simulink model "gm_uz_pmsm_model_9ph_vnl"  (R2021a)
settings: Solver=FixedStepAuto  StartTime=0.0  StopTime=.5  RelTol=1e-3
PreLoadFcn:
  | uz_pmsm_model_init_parameter
undefined symbols (not defined in the file or in its folder): c, friction_coefficient, inertia, k_i_d, k_p_d, k_p_q, L_d, L_o1, L_o2, L_q, L_x1, L_x2, L_y1, L_y2, L_zero, polepair, psi_pm, R_1, static_friction_torque, ts
libraries: hdlmdlgenlib x220, hdlsllib x18, simulink x11, pid_lib x2
(part 3 of 4)

== system gm_uz_pmsm_model_9ph_vnl/uz_pmsm_model_9ph/Data Type Conversion12 ==
  In1 : Inport
  Data Type Conversion12 : DataTypeConversion  OutDataTypeStr=double  RndMeth=Nearest  SampleTime=1e-08
  Out1 : Outport
  wires:
  Data Type Conversion12/1 -> Out1/1
  In1/1 -> Data Type Conversion12/1

== system gm_uz_pmsm_model_9ph_vnl/uz_pmsm_model_9ph/Data Type Conversion13 ==
  In1 : Inport
  Data Type Conversion13 : DataTypeConversion  OutDataTypeStr=double  RndMeth=Nearest  SampleTime=1e-08
  Out1 : Outport
  wires:
  Data Type Conversion13/1 -> Out1/1
  In1/1 -> Data Type Conversion13/1

== system gm_uz_pmsm_model_9ph_vnl/uz_pmsm_model_9ph/Data Type Conversion15 ==
  In1 : Inport
  Data Type Conversion15 : DataTypeConversion  OutDataTypeStr=single  RndMeth=Nearest  SampleTime=1e-08
  Out1 : Outport
  wires:
  Data Type Conversion15/1 -> Out1/1
  In1/1 -> Data Type Conversion15/1

== system gm_uz_pmsm_model_9ph_vnl/uz_pmsm_model_9ph/Data Type Conversion16 ==
  In1 : Inport
  Data Type Conversion16 : DataTypeConversion  OutDataTypeStr=single  RndMeth=Nearest  SampleTime=1e-08
  Out1 : Outport
  wires:
  Data Type Conversion16/1 -> Out1/1
  In1/1 -> Data Type Conversion16/1

== system gm_uz_pmsm_model_9ph_vnl/uz_pmsm_model_9ph/Data Type Conversion17 ==
  In1 : Inport
  Data Type Conversion17 : DataTypeConversion  OutDataTypeStr=single  RndMeth=Nearest  SampleTime=1e-08
  Out1 : Outport
  wires:
  Data Type Conversion17/1 -> Out1/1
  In1/1 -> Data Type Conversion17/1

== system gm_uz_pmsm_model_9ph_vnl/uz_pmsm_model_9ph/Data Type Conversion18 ==
  In1 : Inport
  Data Type Conversion18 : DataTypeConversion  OutDataTypeStr=single  RndMeth=Nearest  SampleTime=1e-08
  Out1 : Outport
  wires:
  Data Type Conversion18/1 -> Out1/1
  In1/1 -> Data Type Conversion18/1

== system gm_uz_pmsm_model_9ph_vnl/uz_pmsm_model_9ph/Data Type Conversion19 ==
  In1 : Inport
  Data Type Conversion19 : DataTypeConversion  OutDataTypeStr=double  RndMeth=Nearest  SampleTime=1e-08
  Out1 : Outport
  wires:
  Data Type Conversion19/1 -> Out1/1
  In1/1 -> Data Type Conversion19/1

== system gm_uz_pmsm_model_9ph_vnl/uz_pmsm_model_9ph/Data Type Conversion2 ==
  In1 : Inport
  Data Type Conversion2 : DataTypeConversion  OutDataTypeStr=double  RndMeth=Nearest  SampleTime=1e-08
  Out1 : Outport
  wires:
  Data Type Conversion2/1 -> Out1/1
  In1/1 -> Data Type Conversion2/1

== system gm_uz_pmsm_model_9ph_vnl/uz_pmsm_model_9ph/Data Type Conversion21 ==
  In1 : Inport
  Data Type Conversion21 : DataTypeConversion  OutDataTypeStr=double  RndMeth=Nearest  SampleTime=1e-08
  Out1 : Outport
  wires:
  Data Type Conversion21/1 -> Out1/1
  In1/1 -> Data Type Conversion21/1

== system gm_uz_pmsm_model_9ph_vnl/uz_pmsm_model_9ph/Data Type Conversion26 ==
  In1 : Inport
  Data Type Conversion26 : DataTypeConversion  OutDataTypeStr=single  RndMeth=Nearest  SampleTime=1e-08
  Out1 : Outport
  wires:
  Data Type Conversion26/1 -> Out1/1
  In1/1 -> Data Type Conversion26/1

== system gm_uz_pmsm_model_9ph_vnl/uz_pmsm_model_9ph/Data Type Conversion3 ==
  In1 : Inport
  Data Type Conversion3 : DataTypeConversion  OutDataTypeStr=double  RndMeth=Nearest  SampleTime=1e-08
  Out1 : Outport
  wires:
  Data Type Conversion3/1 -> Out1/1
  In1/1 -> Data Type Conversion3/1

== system gm_uz_pmsm_model_9ph_vnl/uz_pmsm_model_9ph/Data Type Conversion30 ==
  In1 : Inport
  Data Type Conversion30 : DataTypeConversion  OutDataTypeStr=single  RndMeth=Nearest  SampleTime=1e-08
  Out1 : Outport
  wires:
  Data Type Conversion30/1 -> Out1/1
  In1/1 -> Data Type Conversion30/1

== system gm_uz_pmsm_model_9ph_vnl/uz_pmsm_model_9ph/Data Type Conversion31 ==
  In1 : Inport
  Data Type Conversion31 : DataTypeConversion  OutDataTypeStr=fixdt(1, 25, 12)  RndMeth=Nearest  SampleTime=1e-08
  Out1 : Outport
  wires:
  Data Type Conversion31/1 -> Out1/1
  In1/1 -> Data Type Conversion31/1

== system gm_uz_pmsm_model_9ph_vnl/uz_pmsm_model_9ph/Data Type Conversion32 ==
  In1 : Inport
  Data Type Conversion32 : DataTypeConversion  OutDataTypeStr=double  RndMeth=Nearest  SampleTime=1e-08
  Out1 : Outport
  wires:
  Data Type Conversion32/1 -> Out1/1
  In1/1 -> Data Type Conversion32/1

== system gm_uz_pmsm_model_9ph_vnl/uz_pmsm_model_9ph/Data Type Conversion4 ==
  In1 : Inport
  Data Type Conversion4 : DataTypeConversion  OutDataTypeStr=double  RndMeth=Nearest  SampleTime=1e-08
  Out1 : Outport
  wires:
  Data Type Conversion4/1 -> Out1/1
  In1/1 -> Data Type Conversion4/1

== system gm_uz_pmsm_model_9ph_vnl/uz_pmsm_model_9ph/Data Type Conversion41 ==
  In1 : Inport
  Data Type Conversion41 : DataTypeConversion  OutDataTypeStr=double  RndMeth=Nearest  SampleTime=1e-08
  Out1 : Outport
  wires:
  Data Type Conversion41/1 -> Out1/1
  In1/1 -> Data Type Conversion41/1

== system gm_uz_pmsm_model_9ph_vnl/uz_pmsm_model_9ph/Data Type Conversion5 ==
  In1 : Inport
  Data Type Conversion5 : DataTypeConversion  OutDataTypeStr=double  RndMeth=Nearest  SampleTime=1e-08
  Out1 : Outport
  wires:
  Data Type Conversion5/1 -> Out1/1
  In1/1 -> Data Type Conversion5/1

== system gm_uz_pmsm_model_9ph_vnl/uz_pmsm_model_9ph/Data Type Conversion51 ==
  In1 : Inport
  Data Type Conversion51 : DataTypeConversion  OutDataTypeStr=double  RndMeth=Nearest  SampleTime=1e-08
  Out1 : Outport
  wires:
  Data Type Conversion51/1 -> Out1/1
  In1/1 -> Data Type Conversion51/1

== system gm_uz_pmsm_model_9ph_vnl/uz_pmsm_model_9ph/Data Type Conversion6 ==
  In1 : Inport
  Data Type Conversion6 : DataTypeConversion  OutDataTypeStr=single  RndMeth=Nearest  SampleTime=1e-08
  Out1 : Outport
  wires:
  Data Type Conversion6/1 -> Out1/1
  In1/1 -> Data Type Conversion6/1

== system gm_uz_pmsm_model_9ph_vnl/uz_pmsm_model_9ph/Data Type Conversion61 ==
  In1 : Inport
  Data Type Conversion61 : DataTypeConversion  OutDataTypeStr=double  RndMeth=Nearest  SampleTime=1e-08
  Out1 : Outport
  wires:
  Data Type Conversion61/1 -> Out1/1
  In1/1 -> Data Type Conversion61/1

== system gm_uz_pmsm_model_9ph_vnl/uz_pmsm_model_9ph/Data Type Conversion71 ==
  In1 : Inport
  Data Type Conversion71 : DataTypeConversion  OutDataTypeStr=double  RndMeth=Nearest  SampleTime=1e-08
  Out1 : Outport
  wires:
  Data Type Conversion71/1 -> Out1/1
  In1/1 -> Data Type Conversion71/1

== system gm_uz_pmsm_model_9ph_vnl/uz_pmsm_model_9ph/Data Type Conversion8 ==
  In1 : Inport
  Data Type Conversion8 : DataTypeConversion  OutDataTypeStr=double  RndMeth=Nearest  SampleTime=1e-08
  Out1 : Outport
  wires:
  Data Type Conversion8/1 -> Out1/1
  In1/1 -> Data Type Conversion8/1

== system gm_uz_pmsm_model_9ph_vnl/uz_pmsm_model_9ph/Data Type Conversion9 ==
  In1 : Inport
  Data Type Conversion9 : DataTypeConversion  OutDataTypeStr=double  RndMeth=Nearest  SampleTime=1e-08
  Out1 : Outport
  wires:
  Data Type Conversion9/1 -> Out1/1
  In1/1 -> Data Type Conversion9/1

== system gm_uz_pmsm_model_9ph_vnl/uz_pmsm_model_9ph/Data Type Conversion91 ==
  In1 : Inport
  Data Type Conversion91 : DataTypeConversion  OutDataTypeStr=double  RndMeth=Nearest  SampleTime=1e-08
  Out1 : Outport
  wires:
  Data Type Conversion91/1 -> Out1/1
  In1/1 -> Data Type Conversion91/1

== system gm_uz_pmsm_model_9ph_vnl/uz_pmsm_model_9ph/Divide ==
  In1 : Inport
  In2 : Inport  Port=2
  Divide : Product  Inputs=**  OutDataTypeStr=double  SampleTime=1e-08
  Out1 : Outport
  wires:
  Divide/1 -> Out1/1
  In2/1 -> Divide/2
  In1/1 -> Divide/1

== system gm_uz_pmsm_model_9ph_vnl/uz_pmsm_model_9ph/Divide1 ==
  In1 : Inport
  In2 : Inport  Port=2
  Divide1 : Product  Inputs=*/  OutDataTypeStr=double  SampleTime=1e-08
  Out1 : Outport
  wires:
  Divide1/1 -> Out1/1
  In2/1 -> Divide1/2
  In1/1 -> Divide1/1

== system gm_uz_pmsm_model_9ph_vnl/uz_pmsm_model_9ph/Divide10 ==
  In1 : Inport
  In2 : Inport  Port=2
  Divide10 : Product  Inputs=**  OutDataTypeStr=double  SampleTime=1e-08
  Out1 : Outport
  wires:
  Divide10/1 -> Out1/1
  In2/1 -> Divide10/2
  In1/1 -> Divide10/1

== system gm_uz_pmsm_model_9ph_vnl/uz_pmsm_model_9ph/Divide11 ==
  In1 : Inport
  In2 : Inport  Port=2
  Divide11 : Product  Inputs=*/  OutDataTypeStr=double  SampleTime=1e-08
  Out1 : Outport
  wires:
  Divide11/1 -> Out1/1
  In2/1 -> Divide11/2
  In1/1 -> Divide11/1

== system gm_uz_pmsm_model_9ph_vnl/uz_pmsm_model_9ph/Divide12 ==
  In1 : Inport
  In2 : Inport  Port=2
  Divide12 : Product  Inputs=**  OutDataTypeStr=double  SampleTime=1e-08
  Out1 : Outport
  wires:
  Divide12/1 -> Out1/1
  In2/1 -> Divide12/2
  In1/1 -> Divide12/1

== system gm_uz_pmsm_model_9ph_vnl/uz_pmsm_model_9ph/Divide13 ==
  In1 : Inport
  In2 : Inport  Port=2
  Divide13 : Product  Inputs=*/  OutDataTypeStr=double  SampleTime=1e-08
  Out1 : Outport
  wires:
  Divide13/1 -> Out1/1
  In2/1 -> Divide13/2
  In1/1 -> Divide13/1

== system gm_uz_pmsm_model_9ph_vnl/uz_pmsm_model_9ph/Divide14 ==
  In1 : Inport
  In2 : Inport  Port=2
  Divide14 : Product  Inputs=**  OutDataTypeStr=double  SampleTime=1e-08
  Out1 : Outport
  wires:
  Divide14/1 -> Out1/1
  In2/1 -> Divide14/2
  In1/1 -> Divide14/1

== system gm_uz_pmsm_model_9ph_vnl/uz_pmsm_model_9ph/Divide2 ==
  In1 : Inport
  In2 : Inport  Port=2
  Divide2 : Product  Inputs=**  OutDataTypeStr=double  SampleTime=1e-08
  Out1 : Outport
  wires:
  Divide2/1 -> Out1/1
  In2/1 -> Divide2/2
  In1/1 -> Divide2/1

== system gm_uz_pmsm_model_9ph_vnl/uz_pmsm_model_9ph/Divide3 ==
  In1 : Inport
  In2 : Inport  Port=2
  Divide3 : Product  Inputs=*/  OutDataTypeStr=double  SampleTime=1e-08
  Out1 : Outport
  wires:
  Divide3/1 -> Out1/1
  In2/1 -> Divide3/2
  In1/1 -> Divide3/1

== system gm_uz_pmsm_model_9ph_vnl/uz_pmsm_model_9ph/Divide4 ==
  In1 : Inport
  In2 : Inport  Port=2
  Divide4 : Product  Inputs=**  OutDataTypeStr=double  SampleTime=1e-08
  Out1 : Outport
  wires:
  Divide4/1 -> Out1/1
  In2/1 -> Divide4/2
  In1/1 -> Divide4/1

== system gm_uz_pmsm_model_9ph_vnl/uz_pmsm_model_9ph/Divide5 ==
  In1 : Inport
  In2 : Inport  Port=2
  Divide5 : Product  Inputs=*/  OutDataTypeStr=double  SampleTime=1e-08
  Out1 : Outport
  wires:
  Divide5/1 -> Out1/1
  In2/1 -> Divide5/2
  In1/1 -> Divide5/1

== system gm_uz_pmsm_model_9ph_vnl/uz_pmsm_model_9ph/Divide6 ==
  In1 : Inport
  In2 : Inport  Port=2
  Divide6 : Product  Inputs=**  OutDataTypeStr=double  SampleTime=1e-08
  Out1 : Outport
  wires:
  Divide6/1 -> Out1/1
  In2/1 -> Divide6/2
  In1/1 -> Divide6/1

== system gm_uz_pmsm_model_9ph_vnl/uz_pmsm_model_9ph/Divide7 ==
  In1 : Inport
  In2 : Inport  Port=2
  Divide7 : Product  Inputs=*/  OutDataTypeStr=double  SampleTime=1e-08
  Out1 : Outport
  wires:
  Divide7/1 -> Out1/1
  In2/1 -> Divide7/2
  In1/1 -> Divide7/1

== system gm_uz_pmsm_model_9ph_vnl/uz_pmsm_model_9ph/Divide8 ==
  In1 : Inport
  In2 : Inport  Port=2
  Divide8 : Product  Inputs=**  OutDataTypeStr=double  SampleTime=1e-08
  Out1 : Outport
  wires:
  Divide8/1 -> Out1/1
  In2/1 -> Divide8/2
  In1/1 -> Divide8/1

== system gm_uz_pmsm_model_9ph_vnl/uz_pmsm_model_9ph/Divide9 ==
  In1 : Inport
  In2 : Inport  Port=2
  Divide9 : Product  Inputs=*/  OutDataTypeStr=double  SampleTime=1e-08
  Out1 : Outport
  wires:
  Divide9/1 -> Out1/1
  In2/1 -> Divide9/2
  In1/1 -> Divide9/1

== system gm_uz_pmsm_model_9ph_vnl/uz_pmsm_model_9ph/Factor ==
  In1 : Inport
  In2 : Inport  Port=2
  Factor : Product  Inputs=**  OutDataTypeStr=double  SampleTime=1e-08
  Out1 : Outport
  wires:
  Factor/1 -> Out1/1
  In2/1 -> Factor/2
  In1/1 -> Factor/1

== system gm_uz_pmsm_model_9ph_vnl/uz_pmsm_model_9ph/Gain ==
  In1 : Inport
  In2 : Inport  Port=2
  Gain : Product  Inputs=**  OutDataTypeStr=double  SampleTime=1e-08
  Out1 : Outport
  wires:
  Gain/1 -> Out1/1
  In2/1 -> Gain/2
  In1/1 -> Gain/1

== system gm_uz_pmsm_model_9ph_vnl/uz_pmsm_model_9ph/Gain1 ==
  In1 : Inport
  In2 : Inport  Port=2
  Gain1 : Product  Inputs=**  OutDataTypeStr=double  SampleTime=1e-08
  Out1 : Outport
  wires:
  Gain1/1 -> Out1/1
  In2/1 -> Gain1/2
  In1/1 -> Gain1/1

== system gm_uz_pmsm_model_9ph_vnl/uz_pmsm_model_9ph/Gain10 ==
  In1 : Inport
  In2 : Inport  Port=2
  Gain10 : Product  Inputs=**  OutDataTypeStr=double  SampleTime=1e-08
  Out1 : Outport
  wires:
  Gain10/1 -> Out1/1
  In2/1 -> Gain10/2
  In1/1 -> Gain10/1

== system gm_uz_pmsm_model_9ph_vnl/uz_pmsm_model_9ph/Gain2 ==
  In1 : Inport
  In2 : Inport  Port=2
  Gain2 : Product  Inputs=**  OutDataTypeStr=double  SampleTime=1e-08
  Out1 : Outport
  wires:
  Gain2/1 -> Out1/1
  In2/1 -> Gain2/2
  In1/1 -> Gain2/1

== system gm_uz_pmsm_model_9ph_vnl/uz_pmsm_model_9ph/Gain3 ==
  In1 : Inport
  In2 : Inport  Port=2
  Gain3 : Product  Inputs=**  OutDataTypeStr=double  SampleTime=1e-08
  Out1 : Outport
  wires:
  Gain3/1 -> Out1/1
  In2/1 -> Gain3/2
  In1/1 -> Gain3/1

== system gm_uz_pmsm_model_9ph_vnl/uz_pmsm_model_9ph/Gain4 ==
  In1 : Inport
  In2 : Inport  Port=2
  Gain4 : Product  Inputs=**  OutDataTypeStr=double  SampleTime=1e-08
  Out1 : Outport
  wires:
  Gain4/1 -> Out1/1
  In2/1 -> Gain4/2
  In1/1 -> Gain4/1

== system gm_uz_pmsm_model_9ph_vnl/uz_pmsm_model_9ph/Gain5 ==
  In1 : Inport
  In2 : Inport  Port=2
  Gain5 : Product  Inputs=**  OutDataTypeStr=double  SampleTime=1e-08
  Out1 : Outport
  wires:
  Gain5/1 -> Out1/1
  In2/1 -> Gain5/2
  In1/1 -> Gain5/1

== system gm_uz_pmsm_model_9ph_vnl/uz_pmsm_model_9ph/Gain6 ==
  In1 : Inport
  In2 : Inport  Port=2
  Gain6 : Product  Inputs=**  OutDataTypeStr=double  SampleTime=1e-08
  Out1 : Outport
  wires:
  Gain6/1 -> Out1/1
  In2/1 -> Gain6/2
  In1/1 -> Gain6/1

== system gm_uz_pmsm_model_9ph_vnl/uz_pmsm_model_9ph/Gain7 ==
  In1 : Inport
  In2 : Inport  Port=2
  Gain7 : Product  Inputs=**  OutDataTypeStr=double  SampleTime=1e-08
  Out1 : Outport
  wires:
  Gain7/1 -> Out1/1
  In2/1 -> Gain7/2
  In1/1 -> Gain7/1

== system gm_uz_pmsm_model_9ph_vnl/uz_pmsm_model_9ph/Gain8 ==
  In1 : Inport
  In2 : Inport  Port=2
  Gain8 : Product  Inputs=**  OutDataTypeStr=double  SampleTime=1e-08
  Out1 : Outport
  wires:
  Gain8/1 -> Out1/1
  In2/1 -> Gain8/2
  In1/1 -> Gain8/1

== system gm_uz_pmsm_model_9ph_vnl/uz_pmsm_model_9ph/Gain9 ==
  In1 : Inport
  In2 : Inport  Port=2
  Gain9 : Product  Inputs=**  OutDataTypeStr=double  SampleTime=1e-08
  Out1 : Outport
  wires:
  Gain9/1 -> Out1/1
  In2/1 -> Gain9/2
  In1/1 -> Gain9/1

== system gm_uz_pmsm_model_9ph_vnl/uz_pmsm_model_9ph/Product ==
  In1 : Inport
  In2 : Inport  Port=2
  Product : Product  Inputs=**  OutDataTypeStr=double  SampleTime=1e-08
  Out1 : Outport
  wires:
  Product/1 -> Out1/1
  In2/1 -> Product/2
  In1/1 -> Product/1

== system gm_uz_pmsm_model_9ph_vnl/uz_pmsm_model_9ph/Product1 ==
  In1 : Inport
  In2 : Inport  Port=2
  Product1 : Product  Inputs=**  OutDataTypeStr=double  SampleTime=1e-08
  Out1 : Outport
  wires:
  Product1/1 -> Out1/1
  In2/1 -> Product1/2
  In1/1 -> Product1/1

== system gm_uz_pmsm_model_9ph_vnl/uz_pmsm_model_9ph/Product10 ==
  In1 : Inport
  In2 : Inport  Port=2
  Product10 : Product  Inputs=**  OutDataTypeStr=double  SampleTime=1e-08
  Out1 : Outport
  wires:
  Product10/1 -> Out1/1
  In2/1 -> Product10/2
  In1/1 -> Product10/1

== system gm_uz_pmsm_model_9ph_vnl/uz_pmsm_model_9ph/Product11 ==
  In1 : Inport
  In2 : Inport  Port=2
  Product11 : Product  Inputs=**  OutDataTypeStr=double  SampleTime=1e-08
  Out1 : Outport
  wires:
  Product11/1 -> Out1/1
  In2/1 -> Product11/2
  In1/1 -> Product11/1

== system gm_uz_pmsm_model_9ph_vnl/uz_pmsm_model_9ph/Product12 ==
  In1 : Inport
  In2 : Inport  Port=2
  Product12 : Product  Inputs=**  OutDataTypeStr=double  SampleTime=1e-08
  Out1 : Outport
  wires:
  Product12/1 -> Out1/1
  In2/1 -> Product12/2
  In1/1 -> Product12/1

== system gm_uz_pmsm_model_9ph_vnl/uz_pmsm_model_9ph/Product2 ==
  In1 : Inport
  In2 : Inport  Port=2
  Product2 : Product  Inputs=**  OutDataTypeStr=double  SampleTime=1e-08
  Out1 : Outport
  wires:
  Product2/1 -> Out1/1
  In2/1 -> Product2/2
  In1/1 -> Product2/1

== system gm_uz_pmsm_model_9ph_vnl/uz_pmsm_model_9ph/Product3 ==
  In1 : Inport
  In2 : Inport  Port=2
  Product3 : Product  Inputs=**  OutDataTypeStr=double  SampleTime=1e-08
  Out1 : Outport
  wires:
  Product3/1 -> Out1/1
  In2/1 -> Product3/2
  In1/1 -> Product3/1

== system gm_uz_pmsm_model_9ph_vnl/uz_pmsm_model_9ph/Product4 ==
  In1 : Inport
  In2 : Inport  Port=2
  Product4 : Product  Inputs=**  OutDataTypeStr=double  SampleTime=1e-08
  Out1 : Outport
  wires:
  Product4/1 -> Out1/1
  In2/1 -> Product4/2
  In1/1 -> Product4/1

== system gm_uz_pmsm_model_9ph_vnl/uz_pmsm_model_9ph/Product5 ==
  In1 : Inport
  In2 : Inport  Port=2
  Product5 : Product  Inputs=**  OutDataTypeStr=double  SampleTime=1e-08
  Out1 : Outport
  wires:
  Product5/1 -> Out1/1
  In2/1 -> Product5/2
  In1/1 -> Product5/1

== system gm_uz_pmsm_model_9ph_vnl/uz_pmsm_model_9ph/Product6 ==
  In1 : Inport
  In2 : Inport  Port=2
  Product6 : Product  Inputs=**  OutDataTypeStr=double  SampleTime=1e-08
  Out1 : Outport
  wires:
  Product6/1 -> Out1/1
  In2/1 -> Product6/2
  In1/1 -> Product6/1

== system gm_uz_pmsm_model_9ph_vnl/uz_pmsm_model_9ph/Product7 ==
  In1 : Inport
  In2 : Inport  Port=2
  Product7 : Product  Inputs=**  OutDataTypeStr=double  SampleTime=1e-08
  Out1 : Outport
  wires:
  Product7/1 -> Out1/1
  In2/1 -> Product7/2
  In1/1 -> Product7/1

== system gm_uz_pmsm_model_9ph_vnl/uz_pmsm_model_9ph/Product8 ==
  In1 : Inport
  In2 : Inport  Port=2
  Product8 : Product  Inputs=**  OutDataTypeStr=double  SampleTime=1e-08
  Out1 : Outport
  wires:
  Product8/1 -> Out1/1
  In2/1 -> Product8/2
  In1/1 -> Product8/1

== system gm_uz_pmsm_model_9ph_vnl/uz_pmsm_model_9ph/Product9 ==
  In1 : Inport
  In2 : Inport  Port=2
  Product9 : Product  Inputs=**  OutDataTypeStr=double  SampleTime=1e-08
  Out1 : Outport
  wires:
  Product9/1 -> Out1/1
  In2/1 -> Product9/2
  In1/1 -> Product9/1

== system gm_uz_pmsm_model_9ph_vnl/uz_pmsm_model_9ph/Sign1 ==
  In1 : Inport
  Sign1 : Signum  SampleTime=1e-08
  Out1 : Outport
  wires:
  Sign1/1 -> Out1/1
  In1/1 -> Sign1/1

== system gm_uz_pmsm_model_9ph_vnl/uz_pmsm_model_9ph/Sum ==
  In1 : Inport
  In2 : Inport  Port=2
  Sum : Sum  Inputs=+-  OutDataTypeStr=double  SampleTime=1e-08
  Out1 : Outport
  wires:
  Sum/1 -> Out1/1
  In2/1 -> Sum/2
  In1/1 -> Sum/1

== system gm_uz_pmsm_model_9ph_vnl/uz_pmsm_model_9ph/Sum1 ==
  In1 : Inport
  In2 : Inport  Port=2
  Sum1 : Sum  Inputs=+-  OutDataTypeStr=double  SampleTime=1e-08
  Out1 : Outport
  wires:
  Sum1/1 -> Out1/1
  In2/1 -> Sum1/2
  In1/1 -> Sum1/1

== system gm_uz_pmsm_model_9ph_vnl/uz_pmsm_model_9ph/Sum1_stage2 ==
  In1 : Inport
  In2 : Inport  Port=2
  Sum1_stage2 : Sum  Inputs=+-  OutDataTypeStr=double  SampleTime=1e-08
  Out1 : Outport
  wires:
  Sum1_stage2/1 -> Out1/1
  In2/1 -> Sum1_stage2/2
  In1/1 -> Sum1_stage2/1

== system gm_uz_pmsm_model_9ph_vnl/uz_pmsm_model_9ph/Sum1_stage3 ==
  In1 : Inport
  In2 : Inport  Port=2
  Sum1_stage3 : Sum  Inputs=+-  OutDataTypeStr=double  SampleTime=1e-08
  Out1 : Outport
  wires:
  Sum1_stage3/1 -> Out1/1
  In2/1 -> Sum1_stage3/2
  In1/1 -> Sum1_stage3/1

== system gm_uz_pmsm_model_9ph_vnl/uz_pmsm_model_9ph/Sum2 ==
  In1 : Inport
  In2 : Inport  Port=2
  Sum2 : Sum  Inputs=+-  OutDataTypeStr=double  SampleTime=1e-08
  Out1 : Outport
  wires:
  Sum2/1 -> Out1/1
  In2/1 -> Sum2/2
  In1/1 -> Sum2/1

== system gm_uz_pmsm_model_9ph_vnl/uz_pmsm_model_9ph/Sum3 ==
  In1 : Inport
  In2 : Inport  Port=2
  Sum3 : Sum  OutDataTypeStr=double  SampleTime=1e-08
  Out1 : Outport
  wires:
  Sum3/1 -> Out1/1
  In2/1 -> Sum3/2
  In1/1 -> Sum3/1

== system gm_uz_pmsm_model_9ph_vnl/uz_pmsm_model_9ph/Sum31 ==
  In1 : Inport
  In2 : Inport  Port=2
  Sum31 : Sum  OutDataTypeStr=double  SampleTime=1e-08
  Out1 : Outport
  wires:
  Sum31/1 -> Out1/1
  In2/1 -> Sum31/2
  In1/1 -> Sum31/1

== system gm_uz_pmsm_model_9ph_vnl/uz_pmsm_model_9ph/Sum310 ==
  In1 : Inport
  In2 : Inport  Port=2
  Sum310 : Sum  Inputs=+-  OutDataTypeStr=double  SampleTime=1e-08
  Out1 : Outport
  wires:
  Sum310/1 -> Out1/1
  In2/1 -> Sum310/2
  In1/1 -> Sum310/1

== system gm_uz_pmsm_model_9ph_vnl/uz_pmsm_model_9ph/Sum311 ==
  In1 : Inport
  In2 : Inport  Port=2
  Sum311 : Sum  OutDataTypeStr=double  SampleTime=1e-08
  Out1 : Outport
  wires:
  Sum311/1 -> Out1/1
  In2/1 -> Sum311/2
  In1/1 -> Sum311/1

== system gm_uz_pmsm_model_9ph_vnl/uz_pmsm_model_9ph/Sum32 ==
  In1 : Inport
  In2 : Inport  Port=2
  Sum32 : Sum  OutDataTypeStr=double  SampleTime=1e-08
  Out1 : Outport
  wires:
  Sum32/1 -> Out1/1
  In2/1 -> Sum32/2
  In1/1 -> Sum32/1

== system gm_uz_pmsm_model_9ph_vnl/uz_pmsm_model_9ph/Sum33 ==
  In1 : Inport
  In2 : Inport  Port=2
  Sum33 : Sum  OutDataTypeStr=double  SampleTime=1e-08
  Out1 : Outport
  wires:
  Sum33/1 -> Out1/1
  In2/1 -> Sum33/2
  In1/1 -> Sum33/1

== system gm_uz_pmsm_model_9ph_vnl/uz_pmsm_model_9ph/Sum34 ==
  In1 : Inport
  In2 : Inport  Port=2
  Sum34 : Sum  OutDataTypeStr=double  SampleTime=1e-08
  Out1 : Outport
  wires:
  Sum34/1 -> Out1/1
  In2/1 -> Sum34/2
  In1/1 -> Sum34/1

== system gm_uz_pmsm_model_9ph_vnl/uz_pmsm_model_9ph/Sum35 ==
  In1 : Inport
  In2 : Inport  Port=2
  Sum35 : Sum  OutDataTypeStr=double  SampleTime=1e-08
  Out1 : Outport
  wires:
  Sum35/1 -> Out1/1
  In2/1 -> Sum35/2
  In1/1 -> Sum35/1

== system gm_uz_pmsm_model_9ph_vnl/uz_pmsm_model_9ph/Sum36 ==
  In1 : Inport
  In2 : Inport  Port=2
  Sum36 : Sum  OutDataTypeStr=double  SampleTime=1e-08
  Out1 : Outport
  wires:
  Sum36/1 -> Out1/1
  In2/1 -> Sum36/2
  In1/1 -> Sum36/1

== system gm_uz_pmsm_model_9ph_vnl/uz_pmsm_model_9ph/Sum37 ==
  In1 : Inport
  In2 : Inport  Port=2
  Sum37 : Sum  OutDataTypeStr=double  SampleTime=1e-08
  Out1 : Outport
  wires:
  Sum37/1 -> Out1/1
  In2/1 -> Sum37/2
  In1/1 -> Sum37/1

== system gm_uz_pmsm_model_9ph_vnl/uz_pmsm_model_9ph/Sum38 ==
  In1 : Inport
  In2 : Inport  Port=2
  Sum38 : Sum  OutDataTypeStr=double  SampleTime=1e-08
  Out1 : Outport
  wires:
  Sum38/1 -> Out1/1
  In2/1 -> Sum38/2
  In1/1 -> Sum38/1

== system gm_uz_pmsm_model_9ph_vnl/uz_pmsm_model_9ph/Sum39 ==
  In1 : Inport
  In2 : Inport  Port=2
  Sum39 : Sum  OutDataTypeStr=double  SampleTime=1e-08
  Out1 : Outport
  wires:
  Sum39/1 -> Out1/1
  In2/1 -> Sum39/2
  In1/1 -> Sum39/1

== system gm_uz_pmsm_model_9ph_vnl/uz_pmsm_model_9ph/Sum5 ==
  In1 : Inport
  In2 : Inport  Port=2
  Sum5 : Sum  OutDataTypeStr=double  SampleTime=1e-08
  Out1 : Outport
  wires:
  Sum5/1 -> Out1/1
  In2/1 -> Sum5/2
  In1/1 -> Sum5/1

== system gm_uz_pmsm_model_9ph_vnl/uz_pmsm_model_9ph/Sum_stage2 ==
  In1 : Inport
  In2 : Inport  Port=2
  Sum_stage2 : Sum  Inputs=+-  OutDataTypeStr=double  SampleTime=1e-08
  Out1 : Outport
  wires:
  Sum_stage2/1 -> Out1/1
  In2/1 -> Sum_stage2/2
  In1/1 -> Sum_stage2/1

== system gm_uz_pmsm_model_9ph_vnl/uz_pmsm_model_9ph/Sum_stage3 ==
  In1 : Inport
  In2 : Inport  Port=2
  Sum_stage3 : Sum  OutDataTypeStr=double  SampleTime=1e-08
  Out1 : Outport
  wires:
  Sum_stage3/1 -> Out1/1
  In2/1 -> Sum_stage3/2
  In1/1 -> Sum_stage3/1

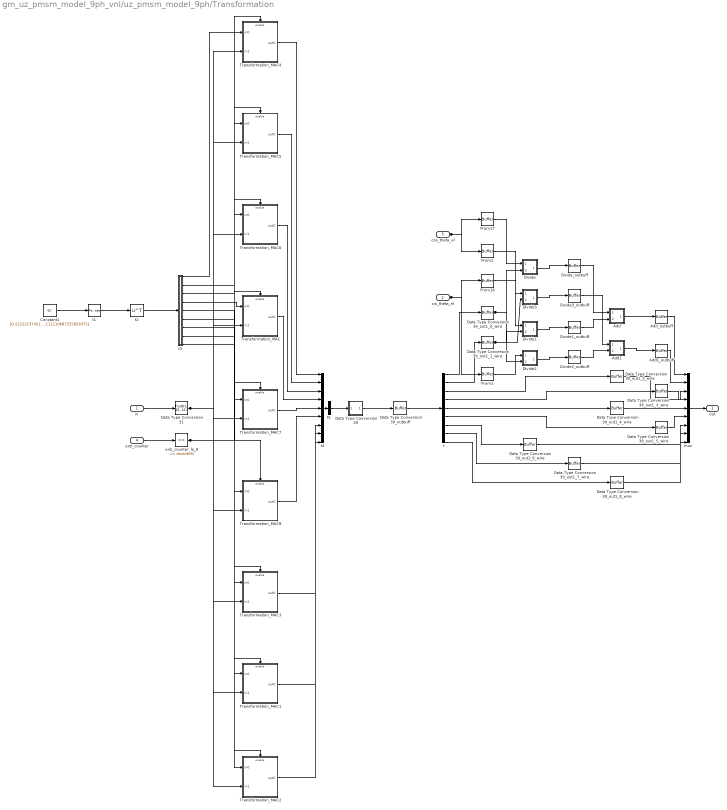
== system gm_uz_pmsm_model_9ph_vnl/uz_pmsm_model_9ph/Transformation ==
  in : Inport  OutDataTypeStr=fixdt(1, 25, 12)  PortDimensions=[9]  SampleTime=1e-08
  sin_theta_el : Inport  Port=2  OutDataTypeStr=single  SampleTime=1e-08
  cos_theta_el : Inport  Port=3  OutDataTypeStr=single  SampleTime=1e-08
  enb_counter : Inport  Port=4  OutDataTypeStr=uint8  SampleTime=1e-08
  Add : Subsystem
      mask Display: disp('NFP\nadd');
  Add1 : Subsystem
      mask Display: disp('NFP\nadd');
  Add1_outbuff : hdlmdlgenlib/Buffer
      settings: SourceProductBaseCode=SL
  Add_outbuff : hdlmdlgenlib/Buffer
      settings: SourceProductBaseCode=SL
  Constant1 : Constant  Value=[0.22222137451171875;0;0.22222137451171875;0;0.22222137451171875;0;0.22222137451171875;0;0.111110687255859375;-0.111110687255859375;0.1924495697021484375;0.22222137451171875;0;-0.111110687255859375;-0.1924495697021484375;-0.111110687255859375;0.1924495697021484375;0.111110687255859375;-0.111110687255859375;-0.1924495697021484375;0.22222137451171875;0;-0.111110687255859375;0.1924495697021484375;-0.111110687255859375;-0.1924495697021484375;0.111110687255859375;0.208820343017578125;0.0760040283203125;0.111110687255859375;0.1924495697021484375;-0.0385875701904296875;0.218845367431640625;-0.1702327728271484375;0.142841339111328125;-0.111110687255859375;-0.1702327728271484375;0.142841339111328125;0.111110687255859375;0.1924495697021484375;0.208820343017578125;-0.0760040283203125;-0.0385875701904296875;-0.218845367431640625;-0.111110687255859375;-0.0385875701904296875;-0.218845367431640625;0.111110687255859375;0.1924495697021484375;-0.1702327728271484375;-0.142841339111328125;0.208820343017578125;0.0760040283203125;-0.111110687255859375;0.1702327728271484375;0.142841339111328125;-0.111110687255859375;0.1924495697021484375;-0.208820343017578125;-0.0760040283203125;0.0385875701904296875;-0.218845367431640625;0.111110687255859375;-0.208820343017578125;0.0760040283203125;-0.111110687255859375;0.1924495697021484375;0.0385875701904296875;0.218845367431640625;0.1702327728271484375;0.142841339111328125;0.111110687255859375;0.0385875701904296875;-0.218845367431640625;-0.111110687255859375;0.1924495697021484375;0.1702327728271484375;-0.142841339111328125;-0.208820343017578125;0.0760040283203125;0.111110687255859375]  OutDataTypeStr=fixdt(1, 18, 19)  SampleTime=1e-08
  Data Type Conversion31 : DataTypeConversion  OutDataTypeStr=fixdt(1, 25, 12)  RndMeth=Nearest  SampleTime=1e-08
  Data Type Conversion39 : Subsystem
      mask Display: disp('NFP\nconv');
  Data Type Conversion39_out1_0_wire : hdlmdlgenlib/Buffer
      settings: SourceProductBaseCode=SL
  Data Type Conversion39_out1_1_wire : hdlmdlgenlib/Buffer
      settings: SourceProductBaseCode=SL
  Data Type Conversion39_out1_2_wire : hdlmdlgenlib/Buffer
      settings: SourceProductBaseCode=SL
  Data Type Conversion39_out1_3_wire : hdlmdlgenlib/Buffer
      settings: SourceProductBaseCode=SL
  Data Type Conversion39_out1_4_wire : hdlmdlgenlib/Buffer
      settings: SourceProductBaseCode=SL
  Data Type Conversion39_out1_5_wire : hdlmdlgenlib/Buffer
      settings: SourceProductBaseCode=SL
  Data Type Conversion39_out1_6_wire : hdlmdlgenlib/Buffer
      settings: SourceProductBaseCode=SL
  Data Type Conversion39_out1_7_wire : hdlmdlgenlib/Buffer
      settings: SourceProductBaseCode=SL
  Data Type Conversion39_out1_8_wire : hdlmdlgenlib/Buffer
      settings: SourceProductBaseCode=SL
  Data Type Conversion39_outbuff : hdlmdlgenlib/Buffer
      settings: SourceProductBaseCode=SL
  Divide : Subsystem
      mask Display: disp('NFP\nmul');
  Divide1 : Subsystem
      mask Display: disp('NFP\nmul');
  Divide1_outbuff : hdlmdlgenlib/Buffer
      settings: SourceProductBaseCode=SL
  Divide2 : Subsystem
      mask Display: disp('NFP\nmul');
  Divide2_outbuff : hdlmdlgenlib/Buffer
      settings: SourceProductBaseCode=SL
  Divide3 : Subsystem
      mask Display: disp('NFP\nmul');
  Divide3_outbuff : hdlmdlgenlib/Buffer
      settings: SourceProductBaseCode=SL
  Divide_outbuff : hdlmdlgenlib/Buffer
      settings: SourceProductBaseCode=SL
  From{1..2,17..18} (4 alike) : hdlmdlgenlib/Buffer
      settings: SourceProductBaseCode=SL
  Transformation_MAC : Subsystem
      settings: MinAlgLoopOccurrences=on
  Transformation_MAC1 : Subsystem
      settings: MinAlgLoopOccurrences=on
  Transformation_MAC2 : Subsystem
      settings: MinAlgLoopOccurrences=on
  Transformation_MAC3 : Subsystem
      settings: MinAlgLoopOccurrences=on
  Transformation_MAC4 : Subsystem
      settings: MinAlgLoopOccurrences=on
  Transformation_MAC5 : Subsystem
      settings: MinAlgLoopOccurrences=on
  Transformation_MAC6 : Subsystem
      settings: MinAlgLoopOccurrences=on
  Transformation_MAC7 : Subsystem
      settings: MinAlgLoopOccurrences=on
  Transformation_MAC8 : Subsystem
      settings: MinAlgLoopOccurrences=on
  enb_counter_le_8 : simulink/Logic and Bit Operations/Compare To Constant  relop=<=  const=double(8)  OutDataTypeStr=boolean
  mux : Mux  Inputs=9
  t : Demux  Outputs=9
  t1 : Reshape  OutputDimensionality=Customize  OutputDimensions=[9,9]
  t2 : Math  Operator=transpose  SaturateOnIntegerOverflow=on
  t3 : Subsystem
  t4 : Mux  Inputs=9
  t5 : Concatenate  NumInputs=1  Mode=Multidimensional array  ConcatenateDimension=2
  out : Outport  SampleTime=1e-08
  wires:
  enb_counter/1 -> enb_counter_le_8/1
  cos_theta_el/1 -> From17/1, From2/1
  sin_theta_el/1 -> From1/1, From18/1
  in/1 -> Data Type Conversion31/1
  enb_counter_le_8/1 -> Transformation_MAC2/Enable, Transformation_MAC1/Enable, Transformation_MAC3/Enable, Transformation_MAC8/Enable, Transformation_MAC7/Enable, Transformation_MAC/Enable, Transformation_MAC6/Enable, Transformation_MAC5/Enable, Transformation_MAC4/Enable
  Divide3/1(Out1) -> Divide3_outbuff/1
  Divide2/1(Out1) -> Divide2_outbuff/1
  Divide1/1(Out1) -> Divide1_outbuff/1
  Divide/1(Out1) -> Divide_outbuff/1
  Data Type Conversion39/1(Out1) -> Data Type Conversion39_outbuff/1
  Add1/1(Out1) -> Add1_outbuff/1
  Add/1(Out1) -> Add_outbuff/1
  From1/1 -> Divide2/1(In1)
  From18/1 -> Divide1/1(In1)
  From2/1 -> Divide3/1(In1)
  From17/1 -> Divide/1(In1)
  t4/1 -> t5/1
  Transformation_MAC2/1(out0) -> t4/9
  Transformation_MAC1/1(out0) -> t4/8
  Transformation_MAC3/1(out0) -> t4/7
  Transformation_MAC8/1(out0) -> t4/6
  Transformation_MAC7/1(out0) -> t4/5
  Transformation_MAC/1(out0) -> t4/4
  Transformation_MAC6/1(out0) -> t4/3
  Transformation_MAC5/1(out0) -> t4/2
  Transformation_MAC4/1(out0) -> t4/1
  t3/9(out8) -> Transformation_MAC2/1(in0)
  t3/8(out7) -> Transformation_MAC1/1(in0)
  t3/7(out6) -> Transformation_MAC3/1(in0)
  t3/6(out5) -> Transformation_MAC8/1(in0)
  t3/5(out4) -> Transformation_MAC7/1(in0)
  t3/4(out3) -> Transformation_MAC/1(in0)
  t3/3(out2) -> Transformation_MAC6/1(in0)
  t3/2(out1) -> Transformation_MAC5/1(in0)
  t3/1(out0) -> Transformation_MAC4/1(in0)
  t2/1 -> t3/1(in0)
  Constant1/1 -> t1/1
  t/9 -> Data Type Conversion39_out1_8_wire/1
  t/8 -> Data Type Conversion39_out1_7_wire/1
  t/7 -> Data Type Conversion39_out1_6_wire/1
  t/6 -> Data Type Conversion39_out1_5_wire/1
  t/5 -> Data Type Conversion39_out1_4_wire/1
  t/4 -> Data Type Conversion39_out1_3_wire/1
  t/3 -> Data Type Conversion39_out1_2_wire/1
  t/2 -> Data Type Conversion39_out1_1_wire/1
  t/1 -> Data Type Conversion39_out1_0_wire/1
  mux/1 -> out/1
  t5/1 -> Data Type Conversion39/1(In1)
  Divide3_outbuff/1 -> Add1/1(In1)
  Divide2_outbuff/1 -> Add1/2(In2)
  Divide1_outbuff/1 -> Add/2(In2)
  Divide_outbuff/1 -> Add/1(In1)
  Data Type Conversion39_out1_8_wire/1 -> mux/9
  Data Type Conversion39_out1_7_wire/1 -> mux/8
  Data Type Conversion39_out1_6_wire/1 -> mux/7
  Data Type Conversion39_out1_5_wire/1 -> mux/6
  Data Type Conversion39_out1_4_wire/1 -> mux/5
  Data Type Conversion39_out1_3_wire/1 -> mux/4
  Data Type Conversion39_out1_2_wire/1 -> mux/3
  Data Type Conversion39_out1_1_wire/1 -> Divide1/2(In2), Divide3/2(In2)
  Data Type Conversion39_out1_0_wire/1 -> Divide/2(In2), Divide2/2(In2)
  Data Type Conversion39_outbuff/1 -> t/1
  Data Type Conversion31/1 -> Transformation_MAC2/2(in1), Transformation_MAC1/2(in1), Transformation_MAC3/2(in1), Transformation_MAC8/2(in1), Transformation_MAC7/2(in1), Transformation_MAC/2(in1), Transformation_MAC6/2(in1), Transformation_MAC5/2(in1), Transformation_MAC4/2(in1)
  t1/1 -> t2/1
  Add1_outbuff/1 -> mux/2
  Add_outbuff/1 -> mux/1

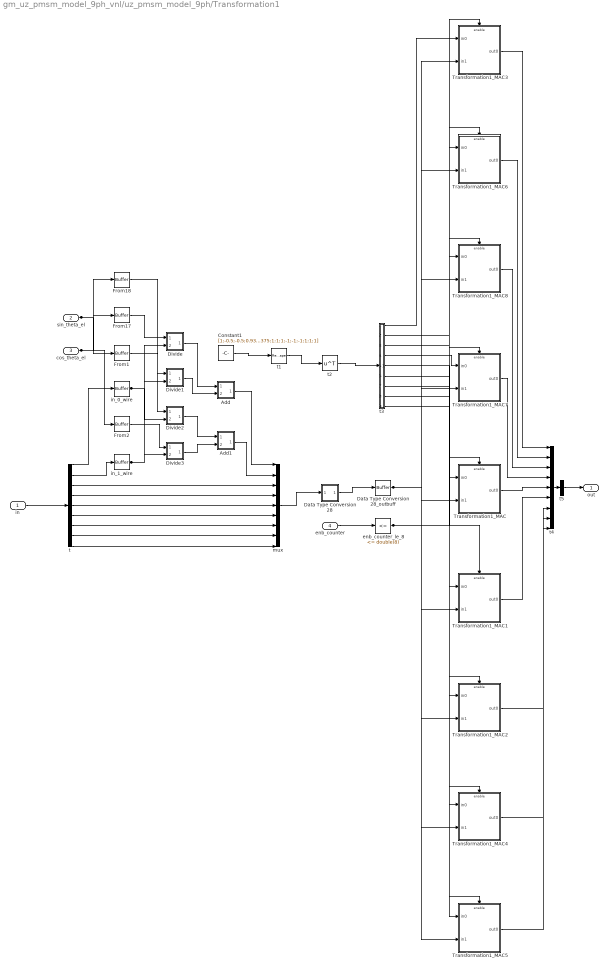
== system gm_uz_pmsm_model_9ph_vnl/uz_pmsm_model_9ph/Transformation1 ==
  in : Inport  OutDataTypeStr=single  PortDimensions=[9]  SampleTime=1e-08
  sin_theta_el : Inport  Port=2  OutDataTypeStr=single  SampleTime=1e-08
  cos_theta_el : Inport  Port=3  OutDataTypeStr=single  SampleTime=1e-08
  enb_counter : Inport  Port=4  OutDataTypeStr=uint8  SampleTime=1e-08
  Add : Subsystem
      mask Display: disp('NFP\nadd');
  Add1 : Subsystem
      mask Display: disp('NFP\nadd');
  Constant1 : Constant  Value=[1;-0.5;-0.5;0.939697265625;-0.7660369873046875;-0.17364501953125;0.7660369873046875;-0.939697265625;0.17364501953125;0;0.86602783203125;-0.86602783203125;0.3420257568359375;0.642791748046875;-0.98480224609375;0.642791748046875;0.3420257568359375;-0.98480224609375;1;1;1;0.5;0.5;0.5;-0.5;-0.5;-0.5;0;0;0;0.86602783203125;0.86602783203125;0.86602783203125;0.86602783203125;0.86602783203125;0.86602783203125;1;-0.5;-0.5;-0.17364501953125;0.939697265625;-0.7660369873046875;-0.939697265625;0.17364501953125;0.7660369873046875;0;-0.86602783203125;0.86602783203125;0.98480224609375;-0.3420257568359375;-0.642791748046875;-0.3420257568359375;0.98480224609375;-0.642791748046875;1;-0.5;-0.5;-0.7660369873046875;-0.17364501953125;0.939697265625;0.17364501953125;0.7660369873046875;-0.939697265625;0;0.86602783203125;-0.86602783203125;0.642791748046875;-0.98480224609375;0.3420257568359375;-0.98480224609375;0.642791748046875;0.3420257568359375;1;1;1;-1;-1;-1;1;1;1]  OutDataTypeStr=fixdt(1, 18, 16)  SampleTime=1e-08
  Data Type Conversion28 : Subsystem
      mask Display: disp('NFP\nconv');
  Data Type Conversion28_outbuff : hdlmdlgenlib/Buffer
      settings: SourceProductBaseCode=SL
  Divide : Subsystem
      mask Display: disp('NFP\nmul');
  Divide1 : Subsystem
      mask Display: disp('NFP\nmul');
  Divide2 : Subsystem
      mask Display: disp('NFP\nmul');
  Divide3 : Subsystem
      mask Display: disp('NFP\nmul');
  From{1..2,17..18} (4 alike) : hdlmdlgenlib/Buffer
      settings: SourceProductBaseCode=SL
  Transformation1_MAC : Subsystem
      settings: MinAlgLoopOccurrences=on
  Transformation1_MAC1 : Subsystem
      settings: MinAlgLoopOccurrences=on
  Transformation1_MAC2 : Subsystem
      settings: MinAlgLoopOccurrences=on
  Transformation1_MAC3 : Subsystem
      settings: MinAlgLoopOccurrences=on
  Transformation1_MAC4 : Subsystem
      settings: MinAlgLoopOccurrences=on
  Transformation1_MAC5 : Subsystem
      settings: MinAlgLoopOccurrences=on
  Transformation1_MAC6 : Subsystem
      settings: MinAlgLoopOccurrences=on
  Transformation1_MAC7 : Subsystem
      settings: MinAlgLoopOccurrences=on
  Transformation1_MAC8 : Subsystem
      settings: MinAlgLoopOccurrences=on
  enb_counter_le_8 : simulink/Logic and Bit Operations/Compare To Constant  relop=<=  const=double(8)  OutDataTypeStr=boolean
  in_0_wire : hdlmdlgenlib/Buffer
      settings: SourceProductBaseCode=SL
  in_1_wire : hdlmdlgenlib/Buffer
      settings: SourceProductBaseCode=SL
  mux : Mux  Inputs=9
  t : Demux  Outputs=9
  t1 : Reshape  OutputDimensionality=Customize  OutputDimensions=[9,9]
  t2 : Math  Operator=transpose  SaturateOnIntegerOverflow=on
  t3 : Subsystem
  t4 : Mux  Inputs=9
  t5 : Concatenate  NumInputs=1  Mode=Multidimensional array  ConcatenateDimension=2
  out : Outport  SampleTime=1e-08
  wires:
  enb_counter/1 -> enb_counter_le_8/1
  cos_theta_el/1 -> From17/1, From2/1
  sin_theta_el/1 -> From1/1, From18/1
  in/1 -> t/1
  enb_counter_le_8/1 -> Transformation1_MAC5/Enable, Transformation1_MAC4/Enable, Transformation1_MAC2/Enable, Transformation1_MAC1/Enable, Transformation1_MAC/Enable, Transformation1_MAC7/Enable, Transformation1_MAC8/Enable, Transformation1_MAC6/Enable, Transformation1_MAC3/Enable
  Divide3/1(Out1) -> Add1/2(In2)
  Divide2/1(Out1) -> Add1/1(In1)
  Divide1/1(Out1) -> Add/2(In2)
  Divide/1(Out1) -> Add/1(In1)
  Data Type Conversion28/1(Out1) -> Data Type Conversion28_outbuff/1
  Add1/1(Out1) -> mux/2
  Add/1(Out1) -> mux/1
  t4/1 -> t5/1
  Transformation1_MAC5/1(out0) -> t4/9
  Transformation1_MAC4/1(out0) -> t4/8
  Transformation1_MAC2/1(out0) -> t4/7
  Transformation1_MAC1/1(out0) -> t4/6
  Transformation1_MAC/1(out0) -> t4/5
  Transformation1_MAC7/1(out0) -> t4/4
  Transformation1_MAC8/1(out0) -> t4/3
  Transformation1_MAC6/1(out0) -> t4/2
  Transformation1_MAC3/1(out0) -> t4/1
  t3/9(out8) -> Transformation1_MAC5/1(in0)
  t3/8(out7) -> Transformation1_MAC4/1(in0)
  t3/7(out6) -> Transformation1_MAC2/1(in0)
  t3/6(out5) -> Transformation1_MAC1/1(in0)
  t3/5(out4) -> Transformation1_MAC/1(in0)
  t3/4(out3) -> Transformation1_MAC7/1(in0)
  t3/3(out2) -> Transformation1_MAC8/1(in0)
  t3/2(out1) -> Transformation1_MAC6/1(in0)
  t3/1(out0) -> Transformation1_MAC3/1(in0)
  t2/1 -> t3/1(in0)
  Constant1/1 -> t1/1
  t/9 -> mux/9
  t/8 -> mux/8
  t/7 -> mux/7
  t/6 -> mux/6
  t/5 -> mux/5
  t/4 -> mux/4
  t/3 -> mux/3
  t/2 -> in_1_wire/1
  t/1 -> in_0_wire/1
  mux/1 -> Data Type Conversion28/1(In1)
  t5/1 -> out/1
  From2/1 -> Divide3/1(In1)
  From18/1 -> Divide1/1(In1)
  From17/1 -> Divide/1(In1)
  From1/1 -> Divide2/1(In1)
  in_1_wire/1 -> Divide1/2(In2), Divide3/2(In2)
  in_0_wire/1 -> Divide/2(In2), Divide2/2(In2)
  Data Type Conversion28_outbuff/1 -> Transformation1_MAC5/2(in1), Transformation1_MAC4/2(in1), Transformation1_MAC2/2(in1), Transformation1_MAC1/2(in1), Transformation1_MAC/2(in1), Transformation1_MAC7/2(in1), Transformation1_MAC8/2(in1), Transformation1_MAC6/2(in1), Transformation1_MAC3/2(in1)
  t1/1 -> t2/1

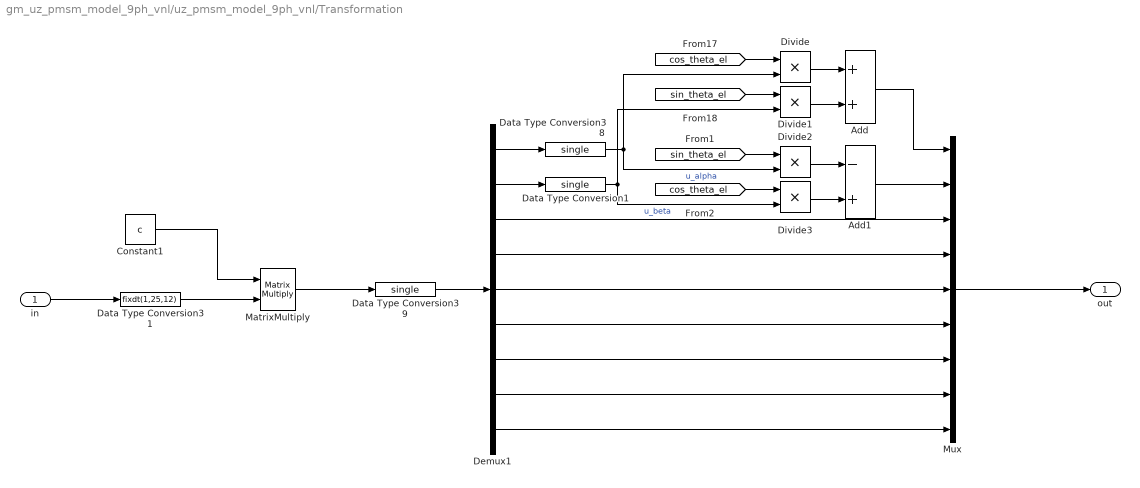
== system gm_uz_pmsm_model_9ph_vnl/uz_pmsm_model_9ph_vnl/Transformation ==
  in : Inport
  Add : Sum
  Add1 : Sum  Inputs=-+
  Constant1 : Constant  Value=c  OutDataTypeStr=fixdt(1,18)  SampleTime=-1
  Data Type Conversion1 : DataTypeConversion  OutDataTypeStr=single  RndMeth=Nearest
  Data Type Conversion31 : DataTypeConversion  OutDataTypeStr=fixdt(1,25,12)  RndMeth=Nearest
  Data Type Conversion38 : DataTypeConversion  OutDataTypeStr=single  RndMeth=Nearest
  Data Type Conversion39 : DataTypeConversion  OutDataTypeStr=single  RndMeth=Nearest
  Demux1 : Demux  Outputs=9
  Divide{,1..3} (4 alike) : Product  Inputs=**
  MatrixMultiply : Product  Multiplication=Matrix(*)
  Mux : Mux  Inputs=9
  out : Outport
  wires:
  Data Type Conversion31/1 -> MatrixMultiply/2
  in/1 -> Data Type Conversion31/1
  Data Type Conversion39/1 -> Demux1/1
  Constant1/1 -> MatrixMultiply/1
  MatrixMultiply/1 -> Data Type Conversion39/1
  Divide2/1 -> Add1/1
  Divide3/1 -> Add1/2
  [cos_theta_el] -> Divide3/1
  [sin_theta_el] -> Divide2/1
  [cos_theta_el] -> Divide/1
  [sin_theta_el] -> Divide1/1
  Divide1/1 -> Add/2
  Divide/1 -> Add/1
  Data Type Conversion1/1 -> Divide3/2, Divide1/2  "u_beta"
  Data Type Conversion38/1 -> Divide2/2, Divide/2  "u_alpha"
  Add/1 -> Mux/1
  Add1/1 -> Mux/2
  Demux1/2 -> Data Type Conversion1/1
  Demux1/1 -> Data Type Conversion38/1
  Mux/1 -> out/1
  Demux1/9 -> Mux/9
  Demux1/8 -> Mux/8
  Demux1/7 -> Mux/7
  Demux1/6 -> Mux/6
  Demux1/5 -> Mux/5
  Demux1/4 -> Mux/4
  Demux1/3 -> Mux/3

== system gm_uz_pmsm_model_9ph_vnl/uz_pmsm_model_9ph_vnl/Transformation1 ==
  in : Inport
  Add : Sum  Inputs=+-
  Add1 : Sum
  Constant1 : Constant  Value=inv(c)  OutDataTypeStr=fixdt(1,18)  SampleTime=-1
  Data Type Conversion28 : DataTypeConversion  OutDataTypeStr=fixdt(1,25,12)  RndMeth=Nearest
  Demux1 : Demux  Outputs=9
  Divide{,1..3} (4 alike) : Product  Inputs=**
  MatrixMultiply : Product  Multiplication=Matrix(*)
  Mux : Mux  Inputs=9
  out : Outport
  wires:
  MatrixMultiply/1 -> out/1
  Constant1/1 -> MatrixMultiply/1
  Data Type Conversion28/1 -> MatrixMultiply/2
  Add1/1 -> Mux/2
  [cos_theta_el] -> Divide3/1
  Divide2/1 -> Add1/1
  [sin_theta_el] -> Divide2/1
  Divide3/1 -> Add1/2
  Demux1/1 -> Divide/2, Divide2/2  "i_d"
  Divide1/1 -> Add/2
  [cos_theta_el] -> Divide/1
  Divide/1 -> Add/1
  Add/1 -> Mux/1
  Demux1/2 -> Divide1/2, Divide3/2  "i_q"
  [sin_theta_el] -> Divide1/1
  Demux1/7 -> Mux/7
  Demux1/9 -> Mux/9
  Demux1/5 -> Mux/5
  Demux1/3 -> Mux/3
  Demux1/4 -> Mux/4
  Demux1/6 -> Mux/6
  Demux1/8 -> Mux/8
  Mux/1 -> Data Type Conversion28/1
  in/1 -> Demux1/1

== system gm_uz_pmsm_model_9ph_vnl/uz_pmsm_model_9ph_vnl/integrator1 ==
  in : Inport
  reset : Inport  Port=2
  Delay1 : Delay  DelayLength=1  ExternalReset=Level
      settings: InputPortMap=u0,r5
  Gain : Gain  Gain=ts  OutDataTypeStr=double
  Sum3 : Sum  Inputs=|++  OutDataTypeStr=double
  outt : Outport
  wires:
  in/1 -> Gain/1
  Gain/1 -> Sum3/1
  reset/1 -> Delay1/2
  Delay1/1 -> Sum3/2, outt/1
  Sum3/1 -> Delay1/1

== system gm_uz_pmsm_model_9ph_vnl/uz_pmsm_model_9ph_vnl/mechanical_system ==
  note: This delay breaks the algebraic loop between mechanical and electrical system.
      | Introduces a delay of 500ns.
  reset : Inport
  M_Mi : Inport  Port=2
  mu : Inport  Port=3
  M_n0 : Inport  Port=4
  reciprocal_J : Inport  Port=5
  load_torque : Inport  Port=6
  Abs : Abs
  Delay : Delay  DelayLength=1
  Product11 : Product
  Product12 : Product
  Product4 : Product
  Sign1 : Signum
  Sum : Sum  Inputs=|+-
  Sum1 : Sum  Inputs=|+-
  Sum5 : Sum  Inputs=|++
  integrator1 : Subsystem
  omega_mech : Outport
  wires:
  Delay/1 -> Sum1/1
  Product4/1 -> Sum/2
  Sum/1 -> Delay/1
  load_torque/1 -> Sum1/2
  Sum1/1 -> Product11/2
  M_Mi/1 -> Sum/1
  reciprocal_J/1 -> Product11/1
  M_n0/1 -> Sum5/2
  mu/1 -> Product12/1
  Product12/1 -> Sum5/1
  reset/1 -> integrator1/1(reset)
  Abs/1 -> Product12/2
  integrator1/1(outt) -> omega_mech/1, Abs/1, Sign1/1
  Sign1/1 -> Product4/2
  Sum5/1 -> Product4/1
  Product11/1 -> integrator1/2(in)

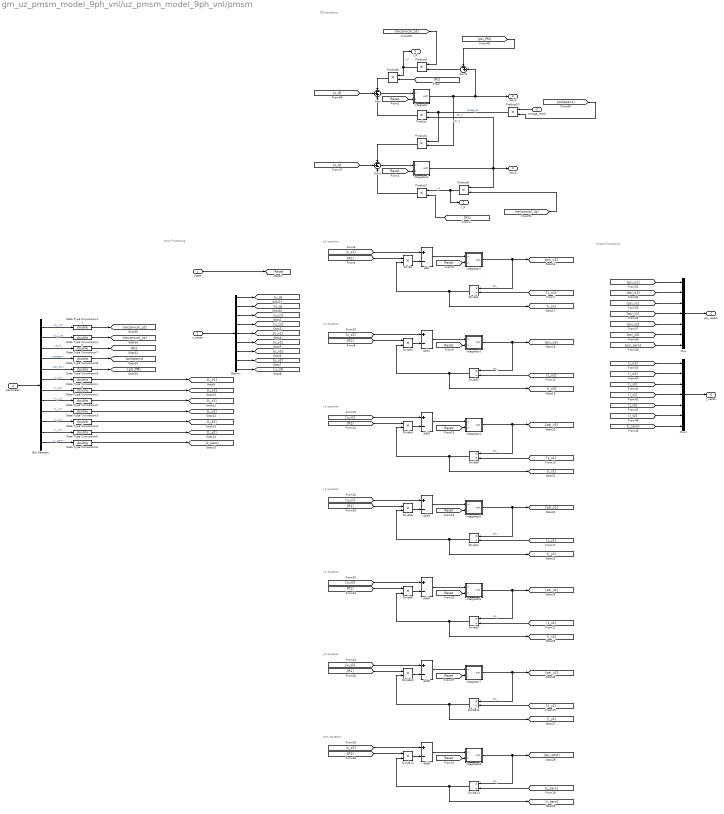
== system gm_uz_pmsm_model_9ph_vnl/uz_pmsm_model_9ph_vnl/pmsm ==
  note: Output Processing
  note: zero equation
  note: y2 equation
  note: x2 equation
  note: y1 equation
  note: x1 equation
  note: o2 equation
  note: DQ equations
  note: o1 equation
  note: Input Processing
  reset : Inport
  u_vector : Inport  Port=2
  omega_mech : Inport  Port=3
  parameter : Inport  Port=4
  Add{,1..6} (7 alike) : Sum  Inputs=+-
  Bus Selector : BusSelector  OutputSignals=1_L_d,1_L_q,R_1,polepair,psi_pm,L_o1,L_o2,L_x1,L_y1,L_x2,L_y2,L_zero
  Data Type Conversion{1..12} (12 alike) : DataTypeConversion  OutDataTypeStr=double  RndMeth=Nearest
  Demux : Demux  Outputs=9
  Divide{,2,4,6,8,10,12} (7 alike) : Product  Inputs=**
  Divide{1,3,5,7,9,11,13} (7 alike) : Product  Inputs=*/
  Mux : Mux  Inputs=7
  Mux1 : Mux  Inputs=7
  Product{,1,5..8,10} (7 alike) : Product
  Sum : Sum  Inputs=-++
  Sum1 : Sum  Inputs=-+-
  Sum2 : Sum  Inputs=-+|
  integrator : Subsystem
  integrator1 : Subsystem
  integrator2 : Subsystem
  integrator3 : Subsystem
  integrator4 : Subsystem
  integrator5 : Subsystem
  integrator6 : Subsystem
  integrator7 : Subsystem
  integrator8 : Subsystem
  I_d : Outport
  I_q : Outport  Port=2
  psi_d : Outport  Port=3
  psi_q : Outport  Port=4
  psi_vector : Outport  Port=5
  I_vector : Outport  Port=6
  tag scope: Reset=global
  wires:
  [R1] -> Divide6/1
  Data Type Conversion11/1 -> [reciprocal_Ld]
  Data Type Conversion12/1 -> [reciprocal_Lq]
  [reciprocal_Lq] -> Product6/2
  Data Type Conversion9/1 -> [psi_PM]
  Data Type Conversion8/1 -> [polepairs]
  Bus Selector/1 -> Data Type Conversion11/1  "<1_L_d>"
  Bus Selector/2 -> Data Type Conversion12/1  "<1_L_q>"
  Bus Selector/5 -> Data Type Conversion9/1  "<psi_pm>"
  Bus Selector/4 -> Data Type Conversion8/1  "<polepair>"
  Data Type Conversion7/1 -> [R1]
  Bus Selector/3 -> Data Type Conversion7/1  "<R_1>"
  Data Type Conversion6/1 -> [L_zero]
  Data Type Conversion5/1 -> [L_y2]
  Data Type Conversion4/1 -> [L_x2]
  Data Type Conversion3/1 -> [L_y1]
  Data Type Conversion2/1 -> [L_x1]
  Data Type Conversion1/1 -> [L_o2]
  Data Type Conversion10/1 -> [L_o1]
  Bus Selector/6 -> Data Type Conversion10/1  "<L_o1>"
  Bus Selector/7 -> Data Type Conversion1/1  "<L_o2>"
  Bus Selector/8 -> Data Type Conversion2/1  "<L_x1>"
  Bus Selector/9 -> Data Type Conversion3/1  "<L_y1>"
  Bus Selector/10 -> Data Type Conversion4/1  "<L_x2>"
  Bus Selector/11 -> Data Type Conversion5/1  "<L_y2>"
  Bus Selector/12 -> Data Type Conversion6/1  "<L_zero>"
  parameter/1 -> Bus Selector/1
  Demux/2 -> [u_q]
  Demux/1 -> [u_d]
  Demux/3 -> [u_z1]
  Demux/4 -> [u_z2]
  Demux/5 -> [u_x1]
  Demux/6 -> [u_y1]
  Demux/7 -> [u_x2]
  Demux/8 -> [u_y2]
  Demux/9 -> [u_z3]
  [i_zero] -> Mux1/7
  [i_y2] -> Mux1/6
  [i_x2] -> Mux1/5
  [i_y1] -> Mux1/4
  [i_x1] -> Mux1/3
  [i_o2] -> Mux1/2
  [psi_zero] -> Mux/7
  [psi_y2] -> Mux/6
  [psi_x2] -> Mux/5
  [psi_y1] -> Mux/4
  [psi_x1] -> Mux/3
  [psi_o2] -> Mux/2
  [i_o1] -> Mux1/1
  [psi_o1] -> Mux/1
  Mux1/1 -> I_vector/1
  Mux/1 -> psi_vector/1
  integrator8/1(outt) -> Divide13/1, [psi_zero]  "psi_"
  [R1] -> Divide12/1
  Add6/1 -> integrator8/1(in)
  Divide12/1 -> Add6/2
  Divide13/1 -> Divide12/2, [i_zero]
  [u_z3] -> Add6/1
  [L_zero] -> Divide13/2
  [Reset] -> integrator8/2(reset)
  [Reset] -> integrator7/2(reset)
  [L_y2] -> Divide11/2
  [u_y2] -> Add5/1
  Divide11/1 -> [i_y2], Divide10/2
  Divide10/1 -> Add5/2
  Add5/1 -> integrator7/1(in)
  [R1] -> Divide10/1
  integrator7/1(outt) -> [psi_y2], Divide11/1  "psi_"
  integrator6/1(outt) -> Divide9/1, [psi_x2]  "psi_"
  [R1] -> Divide8/1
  Add4/1 -> integrator6/1(in)
  Divide8/1 -> Add4/2
  Divide9/1 -> Divide8/2, [i_x2]
  [u_x2] -> Add4/1
  [L_x2] -> Divide9/2
  [Reset] -> integrator6/2(reset)
  [Reset] -> integrator5/2(reset)
  [L_y1] -> Divide7/2
  [u_y1] -> Add3/1
  Divide7/1 -> [i_y1], Divide6/2
  Divide6/1 -> Add3/2
  Add3/1 -> integrator5/1(in)
  integrator5/1(outt) -> [psi_y1], Divide7/1  "psi_"
  integrator4/1(outt) -> Divide5/1, [psi_x1]  "psi_"
  [R1] -> Divide4/1
  Add2/1 -> integrator4/1(in)
  Divide4/1 -> Add2/2
  Divide5/1 -> Divide4/2, [i_x1]
  [u_x1] -> Add2/1
  [L_x1] -> Divide5/2
  [Reset] -> integrator4/2(reset)
  [Reset] -> integrator3/2(reset)
  [L_o2] -> Divide3/2
  [u_z2] -> Add1/1
  Divide3/1 -> [i_o2], Divide2/2
  Divide2/1 -> Add1/2
  Add1/1 -> integrator3/1(in)
  [R1] -> Divide2/1
  integrator3/1(outt) -> [psi_o2], Divide3/1  "psi_"
  integrator2/1(outt) -> Divide1/1, [psi_o1]  "psi_"
  [R1] -> Divide/1
  Add/1 -> integrator2/1(in)
  Divide/1 -> Add/2
  Divide1/1 -> Divide/2, [i_o1]
  [u_z1] -> Add/1
  [L_o1] -> Divide1/2
  [Reset] -> integrator2/2(reset)
  u_vector/1 -> Demux/1
  [Reset] -> integrator1/2(reset)
  [Reset] -> integrator/2(reset)
  reset/1 -> [Reset]
  [R1] -> Product7/2
  [R1] -> Product8/2
  Sum1/1 -> integrator1/1(in)
  Product7/1 -> Sum1/3
  [polepairs] -> Product10/2
  Product8/1 -> Sum/1
  Sum2/1 -> Product5/2
  integrator/1(outt) -> Sum2/2, psi_d/1, Product1/2  "psi_d"
  Product10/1 -> Product/1, Product1/1  "omega_el"
  Product6/1 -> Product7/1, I_q/1  "I_q"
  [psi_PM] -> Sum2/1
  Sum/1 -> integrator/1(in)
  Product1/1 -> Sum1/1
  [u_d] -> Sum/2
  integrator1/1(outt) -> psi_q/1, Product/2, Product6/1  "psi_q"
  [reciprocal_Ld] -> Product5/1
  Product5/1 -> Product8/1, I_d/1  "I_d"
  Product/1 -> Sum/3
  [u_q] -> Sum1/2
  omega_mech/1 -> Product10/1

== system gm_uz_pmsm_model_9ph_vnl/uz_pmsm_model_9ph_vnl/torque_calculation ==
  I_d : Inport
  I_q : Inport  Port=2
  psi_d : Inport  Port=3
  psi_q : Inport  Port=4
  polepairs : Inport  Port=5
  Factor : Gain  Gain=9/2
  Product2 : Product
  Product3 : Product
  Product9 : Product
  Sum3 : Sum  Inputs=-|+
  M_Mi : Outport
  wires:
  Factor/1 -> Product9/1  "M_Mi"
  polepairs/1 -> Product9/2
  Product9/1 -> M_Mi/1  "M_Mi"
  I_q/1 -> Product3/2
  I_d/1 -> Product2/1
  psi_d/1 -> Product3/1
  psi_q/1 -> Product2/2
  Product2/1 -> Sum3/1
  Product3/1 -> Sum3/2
  Sum3/1 -> Factor/1

== system gm_uz_pmsm_model_9ph_vnl/Compare/Assert_output_currents_abc/RelErrCheck ==
  In1 : Inport
  In2 : Inport  Port=2
  "RelativeErrorCheck " : MATLAB Function  TreatAsAtomicUnit=on
  Out1 : Outport  VectorParamsAs1DForOutWhenUnconnected=off
  wires:
  "RelativeErrorCheck "/1(y) -> Out1/1
  In1/1 -> "RelativeErrorCheck "/1(P)
  In2/1 -> "RelativeErrorCheck "/2(R)

== system gm_uz_pmsm_model_9ph_vnl/Compare/Assert_output_currents_dq/RelErrCheck ==
  In1 : Inport
  In2 : Inport  Port=2
  "RelativeErrorCheck " : MATLAB Function  TreatAsAtomicUnit=on
  Out1 : Outport  VectorParamsAs1DForOutWhenUnconnected=off
  wires:
  "RelativeErrorCheck "/1(y) -> Out1/1
  In1/1 -> "RelativeErrorCheck "/1(P)
  In2/1 -> "RelativeErrorCheck "/2(R)

== system gm_uz_pmsm_model_9ph_vnl/Compare/Assert_output_general/RelErrCheck ==
  In1 : Inport
  In2 : Inport  Port=2
  "RelativeErrorCheck " : MATLAB Function  TreatAsAtomicUnit=on
  Out1 : Outport  VectorParamsAs1DForOutWhenUnconnected=off
  wires:
  "RelativeErrorCheck "/1(y) -> Out1/1
  In1/1 -> "RelativeErrorCheck "/1(P)
  In2/1 -> "RelativeErrorCheck "/2(R)

== system gm_uz_pmsm_model_9ph_vnl/uz_pmsm_model_9ph/Transformation/Add ==
  In1 : Inport
  In2 : Inport  Port=2
  Add : Sum  OutDataTypeStr=single  SampleTime=1e-08
  Out1 : Outport
  wires:
  Add/1 -> Out1/1
  In2/1 -> Add/2
  In1/1 -> Add/1

== system gm_uz_pmsm_model_9ph_vnl/uz_pmsm_model_9ph/Transformation/Add1 ==
  In1 : Inport
  In2 : Inport  Port=2
  Add1 : Sum  Inputs=+-  OutDataTypeStr=single  SampleTime=1e-08
  Out1 : Outport
  wires:
  Add1/1 -> Out1/1
  In2/1 -> Add1/2
  In1/1 -> Add1/1

== system gm_uz_pmsm_model_9ph_vnl/uz_pmsm_model_9ph/Transformation/Data Type Conversion39 ==
  In1 : Inport
  Data Type Conversion39 : DataTypeConversion  OutDataTypeStr=single  RndMeth=Nearest  SampleTime=1e-08
  Out1 : Outport
  wires:
  Data Type Conversion39/1 -> Out1/1
  In1/1 -> Data Type Conversion39/1

== system gm_uz_pmsm_model_9ph_vnl/uz_pmsm_model_9ph/Transformation/Divide ==
  In1 : Inport
  In2 : Inport  Port=2
  Divide : Product  Inputs=**  OutDataTypeStr=single  SampleTime=1e-08
  Out1 : Outport
  wires:
  Divide/1 -> Out1/1
  In2/1 -> Divide/2
  In1/1 -> Divide/1

== system gm_uz_pmsm_model_9ph_vnl/uz_pmsm_model_9ph/Transformation/Divide1 ==
  In1 : Inport
  In2 : Inport  Port=2
  Divide1 : Product  Inputs=**  OutDataTypeStr=single  SampleTime=1e-08
  Out1 : Outport
  wires:
  Divide1/1 -> Out1/1
  In2/1 -> Divide1/2
  In1/1 -> Divide1/1
